simulink model "SerialComm"  (R2021a)
settings: Solver=FixedStepAuto  StartTime=0.0  StopTime=10.0  FixedStep=1e-3  RelTol=1e-3  EnableMultiTasking=on
undefined symbols (not defined in the file): A0, A1, D0, D1, D10, D11, D12, D13, D2, D3, D4, D5, D6, D7, D8, D9, magnitude, PTA0, PTA1, PTA2, PTB2, PTB23, PTB3, PTB9, PTC16, PTC17, PTC2, PTC3, PTC4, PTD0, PTD1, PTD2, PTD3
libraries: frdmk64flib x23, etargetslib x6, dspstat3 x1, simulink x1
(part 3 of 3)

== stateflow chart SerialComm/Input Hiding/COM_IN ==
  settings: executeAtInitialization=1
  state ENTRY
    % Initialize Values
    entry:
    LRL = 60000/60;
    AAmplitude = 100;
    APulseW = 10;
    ASensitivity = 80;
    ARP = 250;
    VAmplitude = 100;
    VPulseW = 10;
    VSensitivity = 80;
    VRP = 320;
    AVDelay = 50;
    ActThresh = 1+0*0.4;
    Reaction = 16;
    Response = 10;
    Recovery = 500;
    MSR = 60000/120;
    Mode = 4;
  state SET_VALUES
    % Set Values Through DCM
    entry:
    LRL = 60000/uint16(RxData(3));
    AAmplitude = RxData(4);
    APulseW = RxData(5);
    ASensitivity = RxData(6);
    ARP = typecast(RxData(7:8),'uint16');
    VAmplitude = RxData(9);
    VPulseW = RxData(10);
    VSensitivity = RxData(11);
    VRP = typecast(RxData(12:13),'uint16');
    AVDelay = typecast(RxData(14:15),'uint16');
    ActThresh = 1+double(RxData(16))*0.4;
    Reaction = RxData(17);
    Response = RxData(18);
    Recovery = typecast(RxData(19:20),'uint16');
    MSR = 60000/uint16(RxData(21));
    Mode = RxData(22) + 1;
  note: Set values if
      | first 2 RxData
      | bytes are 12, 5
  note: Set initial
      | values upon
      | entry
  state STANDBY
    %Wait for data
  note: Check if all bytes have been received
  state SEND_PARAMETER
    entry: send_data();
  note: Send data if first 2 RxData bytes are 12, 15
  SET_VALUES -> STANDBY
  (default) -> ENTRY
  ENTRY -> STANDBY
  (junction 77) -> SET_VALUES [order 1] : [RxData(2) == 5]
      | {Mode = 0;}
  (junction 77) -> STANDBY [order 3]
  STANDBY -> (junction 77) : [Status == 0 && length(RxData) == 22 && RxData(1) == 12]
  (junction 77) -> SEND_PARAMETER [order 2] : [RxData(2) == 15]
  SEND_PARAMETER -> STANDBY
  data: LRL output uint16; AAmplitude output uint8; APulseW output uint8; ASensitivity output uint8; ARP output uint16; VAmplitude output uint8; VPulseW output uint8; VSensitivity output uint8; VRP output uint16; AVDelay output uint16; ActThresh output double; Reaction output uint8; Response output uint8; Recovery output uint16; MSR output uint16; RxData input uint8; Status input uint8; Mode output uint8
